simulink model "Drawing_Block"  (R2019a)
settings: Solver=VariableStepAuto  StartTime=0.0  StopTime=40  RelTol=1e-3
settings Model: Creator=Leonard  LastModifiedBy=Leonard

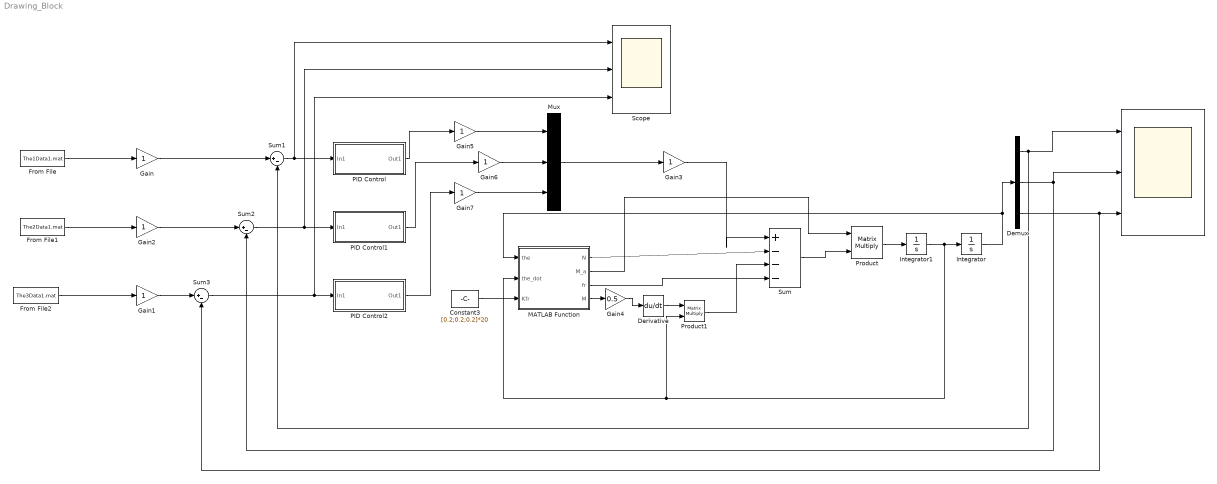
== system Drawing_Block ==
  " " : Scope  NumInputPorts=3
  Constant3 : Constant  Value=[0.2;0.2;0.2]*20
  Demux : Demux  Outputs=3
  Derivative : Derivative
  From File : FromFile  FileName=The1Data1.mat  SampleTime=0
  From File1 : FromFile  FileName=The2Data1.mat  SampleTime=0
  From File2 : FromFile  FileName=The3Data1.mat  SampleTime=0
  Gain{,1..3,5..7} (7 alike) : Gain
  Gain4 : Gain  Gain=0.5
  Integrator : Integrator  InitialCondition=[0;0;0]
  Integrator1 : Integrator  InitialCondition=[0;0;0]
  MATLAB Function : MATLAB Function  TreatAsAtomicUnit=on
  Mux : Mux  Inputs=3
  PID Control : Subsystem
  PID Control1 : Subsystem
  PID Control2 : Subsystem
  Product : Product  Multiplication=Matrix(*)
  Product1 : Product  Multiplication=Matrix(*)
  Scope : Scope  NumInputPorts=3
  Sum : Sum  Inputs=|+---
  Sum1 : Sum  Inputs=|+-
  Sum2 : Sum  Inputs=|+-
  Sum3 : Sum  Inputs=|+-
  wires:
  From File/1 -> Gain/1
  Gain6/1 -> Mux/2
  PID Control/1(Out1) -> Gain5/1
  Demux/1 -> Sum1/2, " "/1
  Demux/3 -> Sum3/2, " "/3
  Product1/1 -> Sum/3
  PID Control2/1(Out1) -> Gain7/1
  Constant3/1 -> MATLAB Function/3(Kfr)
  Gain1/1 -> Sum3/1
  Gain/1 -> Sum1/1
  PID Control1/1(Out1) -> Gain6/1
  Gain7/1 -> Mux/3
  Sum/1 -> Product/2
  Demux/2 -> " "/2, Sum2/2
  MATLAB Function/4(M) -> Gain4/1
  Gain2/1 -> Sum2/1
  From File1/1 -> Gain2/1
  Sum1/1 -> PID Control/1(In1), Scope/1
  Integrator1/1 -> Product1/2, MATLAB Function/2(the_dot), Integrator/1
  Derivative/1 -> Product1/1
  MATLAB Function/2(M_a) -> Product/1
  Sum2/1 -> PID Control1/1(In1), Scope/2
  Integrator/1 -> MATLAB Function/1(the), Demux/1
  Gain4/1 -> Derivative/1
  MATLAB Function/1(N) -> Sum/2
  MATLAB Function/3(fr) -> Sum/4
  Gain3/1 -> Sum/1
  Mux/1 -> Gain3/1
  Gain5/1 -> Mux/1
  From File2/1 -> Gain1/1
  Product/1 -> Integrator1/1
  Sum3/1 -> Scope/3, PID Control2/1(In1)

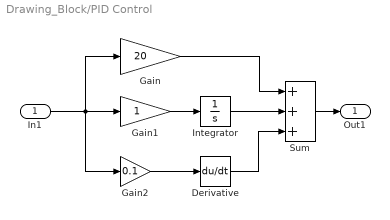
== system Drawing_Block/PID Control ==
  In1 : Inport
  Derivative : Derivative
  Gain : Gain  Gain=20
  Gain1 : Gain
  Gain2 : Gain  Gain=0.1
  Integrator : Integrator
  Sum : Sum  Inputs=+++
  Out1 : Outport
  wires:
  Sum/1 -> Out1/1
  Gain/1 -> Sum/1
  Gain2/1 -> Derivative/1
  Gain1/1 -> Integrator/1
  Integrator/1 -> Sum/2
  Derivative/1 -> Sum/3
  In1/1 -> Gain1/1, Gain2/1, Gain/1

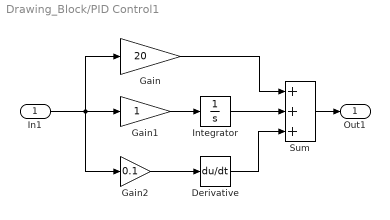
== system Drawing_Block/PID Control1 ==
  In1 : Inport
  Derivative : Derivative
  Gain : Gain  Gain=20
  Gain1 : Gain
  Gain2 : Gain  Gain=0.1
  Integrator : Integrator
  Sum : Sum  Inputs=+++
  Out1 : Outport
  wires:
  Sum/1 -> Out1/1
  Gain/1 -> Sum/1
  Gain2/1 -> Derivative/1
  Gain1/1 -> Integrator/1
  Integrator/1 -> Sum/2
  Derivative/1 -> Sum/3
  In1/1 -> Gain1/1, Gain2/1, Gain/1

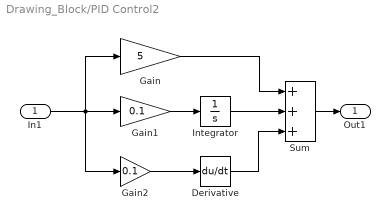
== system Drawing_Block/PID Control2 ==
  In1 : Inport
  Derivative : Derivative
  Gain : Gain  Gain=5
  Gain1 : Gain  Gain=0.1
  Gain2 : Gain  Gain=0.1
  Integrator : Integrator
  Sum : Sum  Inputs=+++
  Out1 : Outport
  wires:
  Sum/1 -> Out1/1
  Gain/1 -> Sum/1
  Gain2/1 -> Derivative/1
  Gain1/1 -> Integrator/1
  Integrator/1 -> Sum/2
  Derivative/1 -> Sum/3
  In1/1 -> Gain1/1, Gain2/1, Gain/1

== matlab function Drawing_Block/MATLAB Function ==
  data: the input; N output; M_a output; fr output; M output; the_dot input; Kfr input
function [N,M_a,fr,M] = fcn(the,the_dot,Kfr)
the1=the(1); the2=the(2); the3=the(3);
L1 = 0.2; L2 = 0.5 ; L3= 0.5; %Link length
m1 = 2 ; m2 = 0.3 ; m3 =0.1 ; %Link mass
%clc
%clear all;
%syms m1 m2 m3 L2 L3 the1 the2 the3 L1 the1_dot the2_dot the3_dot ;
%the_dot = [the1_dot; the2_dot;the3_dot];
%%%%%%%%%%%%%%%%%%%%%%%%%%%%%%%%%%%%%

%TINH JACOBIAN CHO DIEM m1
%P_0_m1 = [ 0; 0; L1];

%DAO HAM P_0_m1 THEO THE1
J_0_m1_dot_the1 = [ 0; 0; 0];
%DAO HAM P_0_m1 THEO THE2
J_0_m1_dot_the2 = [ 0; 0; 0];
%DAO HAM P_0_m1 THEO THE3
J_0_m1_dot_the3 = [ 0; 0; 0]; 

J_0_m1 = [J_0_m1_dot_the1 J_0_m1_dot_the2 J_0_m1_dot_the3];
%%%%%%%%%%%%%%%%%%%%%%%%%%%%%%%%%%%%%%%
%TINH JACOBIAN CHO DIEM m2
%P_0_m2 = [L2*cos(the1)*cos(the2); L2*cos(the2)*sin(the1); L1 + L2*sin(the2)];

%DAO HAM P_0_m2 THEO THE1
J_0_m2_dot_the1 = [L2*sin(-the1)*cos(the2);L2*cos(the2)*cos(the1); 0];
%DAO HAM P_0_m2 THEO THE2
J_0_m2_dot_the2 = [L2*cos(the1)*sin(-the2);L2*sin(-the2)*sin(the1); L2*cos(the2)];
%DAO HAM P_0_m2 THEO THE3
J_0_m2_dot_the3 = [ 0; 0; 0]; 

J_0_m2 = [J_0_m2_dot_the1  J_0_m2_dot_the2  J_0_m2_dot_the3];
%%%%%%%%%%%%%%%%%%%%%%%%%%%%%%%%%%%%%%%%%

%TINH JACOBIAN CHO DIEM m3
%P_0_m3 = [ cos(the1)*(L3*cos(the2 + the3) + L2*cos(the2)); sin(the1)*(L3*cos(the2 + the3) + L2*cos(the2)); L1 + L3*sin(the2 + the3) + L2*sin(the2)];
%DAO HAM P_0_m3 THEO THE1
J_0_m3_dot_the1 = [sin(-the1)*(L3*cos(the2 + the3) + L2*cos(the2));	 cos(the1)*(L3*cos(the2 + the3) + L2*cos(the2));     0];
%DAO HAM P_0_m3 THEO THE2
J_0_m3_dot_the2 = [cos(the1)*(L3*sin(-the2 - the3) + L2*sin(-the2));  sin(the1)*(L3*sin(-the2 - the3) + L2*sin(-the2));    L3*cos(the2 + the3) + L2*cos(the2)];
%DAO HAM P_0_m3 THEO THE3
J_0_m3_dot_the3 = [ cos(the1)*L3*sin(-the2 - the3);	 sin(the1)*L3*sin(-the2 - the3);  L3*cos(the2 + the3)];

J_0_m3 = [J_0_m3_dot_the1  J_0_m3_dot_the2  J_0_m3_dot_the3];

%%%%%%%%%%%%%%%%%%%%%%%%%%%%%%%%%%%%%%%%%%%%%%%%%%%%%%%%%%
%TONG HOP MA TRAN M3

M3 = (m3*[0 0 1]*transpose(J_0_m3)*J_0_m3)

%%%%%%%%%%%%%%%%%%%%%%%%%%%%%%%%%%%%%%%%%%%%%%%%%%%
%TONG HOP MA TRAN M2

M2 = (m2*[0 1 0]*transpose(J_0_m2)*J_0_m2 + m3*[0 1 0]*transpose(J_0_m3)*J_0_m3) 

%%%%%%%%%%%%%%%%%%%%%%%%%%%%%%%%%%%%%%%%%%%%%%%%%%%
%TONG HOP MA TRAN M1

M1 = (m1*[1 0 0]*transpose(J_0_m1)*J_0_m1 + m2*[1 0 0]*transpose(J_0_m2)*J_0_m2 + m3*[1 0 0]*transpose(J_0_m2)*J_0_m3) + [0.1 0 0];


M  = [ M1 ; M2 ; M3];
M_a = inv(M);


%%%%%%%%%%%%%%%%%%%%%%%%%%%%%%%%%%%%%%%%%%%%%%%%%%%%%%
 
%DAO HAM J_0_m1_dot_the1 theo the1

J_0_m1_dot_the1_dot_the1 = [ 0; 0; 0];
%DAO HAM J_0_m1_dot_the2 theo the1
J_0_m1_dot_the2_dot_the1 = [ 0; 0; 0];  
%DAO HAM J_0_m1_dot_the3 theo the1
J_0_m1_dot_the3_dot_the1 = [ 0; 0; 0]; 

%DAO HAM J_0_m1 theo the1 
J_0_m1_dot_the1_1 = [J_0_m1_dot_the1_dot_the1  J_0_m1_dot_the2_dot_the1  J_0_m1_dot_the3_dot_the1];

%%%%%%%%%%%%%%%%%%%%%%%%%%%%%%%%%%%%%%%%%%%%%%%%%%%%%%%%%%
%DAO HAM J_0_m2_dot_the1 theo the1
%J_0_m2_dot_the1 = [L2*sin(-the1)*cos(the2);    L2*cos(the2)*cos(the1);  0];
J_0_m2_dot_the1_dot_the1 = [L2*cos(the1)*cos(the2);L2*cos(the2)*sin(-the1); 0];
%DAO HAM J_0_m2_dot_the2 theo the1
%J_0_m2_dot_the2 = [L2*cos(the1)*sin(-the2);    L2*sin(-the2)*sin(the1);     L2*cos(the2)];
J_0_m2_dot_the2_dot_the1 = [L2*sin(the1)*sin(the2);L2*sin(-the2)*cos(the1); 0];
%DAO HAM J_0_m2_dot_the3 theo the1
J_0_m2_dot_the3_dot_the1 = [ 0; 0; 0]; 

%DAO HAM J_0_m2 theo the1 
J_0_m2_dot_the1_1 = [J_0_m2_dot_the1_dot_the1   J_0_m2_dot_the2_dot_the1  J_0_m2_dot_the3_dot_the1];

%%%%%%%%%%%%%%%%%%%%%%%%%%%%%%%%%%%%%%%%%%%%%%%%%%%%%%%%%%%
%DAO HAM J_0_m2_dot_the1 theo the2
%J_0_m2_dot_the1 = [L2*sin(-the1)*cos(the2);    L2*cos(the2)*cos(the1);  0];
J_0_m2_dot_the1_dot_the2 = [L2*sin(the1)*sin(the2);L2*sin(-the2)*cos(the1); 0];
%DAO HAM J_0_m2_dot_the2 theo the2
%J_0_m2_dot_the2 = [L2*cos(the1)*sin(-the2);    L2*sin(-the2)*sin(the1);     L2*cos(the2)];
J_0_m2_dot_the2_dot_the2 = [L2*cos(the1)*cos(the2);L2*cos(the2)*sin(the1); L2*sin(-the2)];
%DAO HAM J_0_m2_dot_the3 theo the2
J_0_m2_dot_the3_dot_the2 = [ 0; 0; 0]; 

%DAO HAM J_0_m2 theo the2
J_0_m2_dot_the2_2 = [J_0_m2_dot_the1_dot_the2  J_0_m2_dot_the2_dot_the2  J_0_m2_dot_the3_dot_the2];

%%%%%%%%%%%%%%%%%%%%%%%%%%%%%%%%%%%%%%%%%%%%%%%%%%%%%%%%%%%%%%%
%DAO HAM J_0_m3_dot_the1 theo the1
%J_0_m3_dot_the1 = [sin(-the1)*(L3*cos(the2 + the3) + L2*cos(the2));	 cos(the1)*(L3*cos(the2 + the3) + L2*cos(the2));     0];
J_0_m3_dot_the1_dot_the1 = [cos(the1)*(L3*cos(the2 + the3) + L2*cos(the2));	 sin(-the1)*(L3*cos(the2 + the3) + L2*cos(the2));     0];
%DAO HAM J_0_m3_dot_the2 theo the1
%J_0_m3_dot_the2 =          [cos(the1)*(L3*sin(-the2 - the3) + L2*sin(-the2));  sin(the1)*(L3*sin(-the2 - the3) + L2*sin(-the2));    L3*cos(the2 + the3) + L2*cos(the2)];
J_0_m3_dot_the2_dot_the1 = [sin(the1)*(L3*sin(the2 + the3) + L2*sin(the2));  -cos(the1)*(L3*sin(the2 + the3) + L2*sin(the2));    0];
%DAO HAM J_0_m3_dot_the3 theo the1
%J_0_m3_dot_the3 =          [ cos(the1)*L3*sin(-the2 - the3);	 sin(the1)*L3*sin(-the2 - the3);  L3*cos(the2 + the3)];
J_0_m3_dot_the3_dot_the1 = [ sin(the1)*L3*sin(the2 + the3);     -cos(the1)*L3*sin(the2 + the3);  0];

J_0_m3_dot_the1_1 = [J_0_m3_dot_the1_dot_the1  J_0_m3_dot_the2_dot_the1  J_0_m3_dot_the3_dot_the1];

%%%%%%%%%%%%%%%%%%%%%%%%%%%%%%%%%%%%%%%%%%%%%%%%%%%%%%%%%%%%%

%DAO HAM J_0_m3_dot_the1 theo the2
%J_0_m3_dot_the1 =          [sin(-the1)*(L3*cos(the2 + the3) + L2*cos(the2));	 cos(the1)*(L3*cos(the2 + the3) + L2*cos(the2));     0];
J_0_m3_dot_the1_dot_the2 = [sin(the1)*(L3*sin(the2 + the3) + L2*sin(the2));	 -cos(the1)*(L3*sin(the2 + the3) + L2*sin(the2));     0];
%DAO HAM J_0_m3_dot_the2 theo the2
%J_0_m3_dot_the2 =        [cos(the1)*(L3*sin(-the2 - the3) + L2*sin(-the2));  sin(the1)*(L3*sin(-the2 - the3) + L2*sin(-the2));    L3*cos(the2 + the3) + L2*cos(the2)];
J_0_m3_dot_the2_dot_the2 = [cos(the1)*(L3*cos(the2 + the3) + L2*cos(the2));  sin(the1)*(L3*cos(the2 + the3) + L2*cos(the2));    -L3*sin(the2 + the3) - L2*sin(the2)];
%DAO HAM J_0_m3_dot_the3 theo the2
%J_0_m3_dot_the3 =         [ cos(the1)*L3*sin(-the2 - the3);	 sin(the1)*L3*sin(-the2 - the3);  L3*cos(the2 + the3)];
J_0_m3_dot_the3_dot_the2 = [ cos(the1)*L3*cos(the2 + the3);     sin(the1)*L3*cos(the2 + the3);  -L3*sin(the2 + the3)];

%DAO HAM J_0_m3 theo the2
J_0_m3_dot_the2_2= [J_0_m3_dot_the1_dot_the2  J_0_m3_dot_the2_dot_the2  J_0_m3_dot_the3_dot_the2];
 

%%%%%%%%%%%%%%%%%%%%%%%%%%%%%%%%%%%%%%%%%%%%%%%%%%%%%%%%%%%%%
%DAO HAM J_0_m3_dot_the1 theo the3
%J_0_m3_dot_the1 =         [sin(-the1)*(L3*cos(the2 + the3) + L2*cos(the2));	 cos(the1)*(L3*cos(the2 + the3) + L2*cos(the2));     0];
J_0_m3_dot_the1_dot_the3 = [sin(the1)*L3*sin(the2 + the3);	 -cos(the1)*L3*sin(the2 + the3);     0];
%DAO HAM J_0_m3_dot_the2 theo the3
%J_0_m3_dot_the2 =        [cos(the1)*(L3*sin(-the2 - the3) + L2*sin(-the2));  sin(the1)*(L3*sin(-the2 - the3) + L2*sin(-the2));    L3*cos(the2 + the3) + L2*cos(the2)];
J_0_m3_dot_the2_dot_the3 = [cos(the1)*L3*cos(the2 + the3);  sin(the1)*L3*cos(the2 + the3);    -L3*sin(the2 + the3)];
%DAO HAM J_0_m3_dot_the3 theo the3
%J_0_m3_dot_the3 =         [ cos(the1)*L3*sin(-the2 - the3);	 sin(the1)*L3*sin(-the2 - the3);  L3*cos(the2 + the3)];
J_0_m3_dot_the3_dot_the3 = [ cos(the1)*L3*cos(the2 + the3);	 sin(the1)*L3*cos(the2 + the3);  -L3*sin(the2 + the3)];

%DAO HAM J_0_m3 theo the3
J_0_m3_dot_the3_3 = [J_0_m3_dot_the1_dot_the3 J_0_m3_dot_the2_dot_the3  J_0_m3_dot_the3_dot_the3];
 
%%%%%%%%%%%%%%%%%%%%%%%%%%%%%%%%%%%%%%%%%%%%%%%%%%%%%%%%%%%%%%%%%
dT_dthe3 = transpose(the_dot)*(m3*transpose(J_0_m3_dot_the3_3)*J_0_m3)*the_dot;
%%%%%%%%%%%%%%%%%%%%%%%%%%%%%%%%%%%%%%%%%%%%
dT_dthe2 = transpose(the_dot)*(m2*transpose(J_0_m2_dot_the2_2)*J_0_m2+m3*transpose(J_0_m3_dot_the2_2)*J_0_m3)*the_dot;
%%%%%%%%%%%%%%%%%%%%%%%%%%%%%%%%%%%%%%%%%%
dT_dthe1 = (transpose(the_dot)*(m1*transpose(J_0_m1_dot_the1_1)*J_0_m1+m2*transpose(J_0_m2_dot_the1_1)*J_0_m2+m3*transpose(J_0_m3_dot_the1_1)*J_0_m3)*the_dot);

%%%%%%%%%%%%%%%%%%%%%%%%%%%%%%%%%%%%%%%%%%%%%%%%%%%%%%%%%%%%%%%%%%
%M3_dot_t = [ 0,	 (L3*m3*L2*sin(-the3))*the3_dot,	 0];
%M2_dot_t = [ 0, (2*L2*L3*m3*sin(-the3))*the3_dot, 	(L3*m3*L2*sin(-the3))*the3_dot];
%M1_dot_t = [ (2*L2^2*m2*cos(the2)*sin(-the2) + 2*L2^2*m3*cos(the2)*sin(-the2) + 2*L2*L3*m3*cos(the2)*sin(-the2)*cos(the3) - L2*L3*m3*sin(-the2)*cos(the2)*sin(the3))*the2_dot + (L2*L3*m3*cos(the2)^2*sin(-the3) - L2*L3*m3*cos(the2)*sin(the2)*cos(the3))*the3_dot,	 0,	0];

%M_dot_t = [ M1_dot_t;M2_dot_t;M3_dot_t];


%%%%%%%%%%%%%%%%%%%%%%%%%%%%%%%%%%%%%%%%%%%%%%%%%%%%%%%%%
%TINH dU_DTHE3
%%%%%%%%%%%%%%%%%%%%%%%%%%%%%%%%%%%%%%%%%%%%%%%%%%%%%%%%%%%%%%%
g_0 = [ 0;0;-9.81];

dU_dthe3 = -m3*transpose(g_0)*J_0_m3_dot_the3
 
N3 = -dT_dthe3 + dU_dthe3;
%V3 = simplify(-dT_dthe3+M3_dot_t*the_dot)
%%%%%%%%%%%%%%%%%%%%%%%%%%%%%%%%%%%%%%%%%%%%%%%%%%%%%%%%%%%
%TINH dU_DTHE2
%%%%%%%%%%%%%%%%%%%%%%%%%%%%%%%%%%%%%%%%%%%%%%%%%%%%%%%%%%%%%%%
g_0 = [ 0;0;-9.81];

dU_dthe2 = -m2*transpose(g_0)*J_0_m2_dot_the2 - m3*transpose(g_0)*J_0_m3_dot_the2
 
N2= -dT_dthe2 + dU_dthe2;
%V2 = simplify(-dT_dthe2 + M2_dot_t*the_dot)
%%%%%%%%%%%%%%%%%%%%%%%%%%%%%%%%%%%%%%%%%%%%%%%%%%%%%%%%%%%
%TINH dU_DTHE1
%%%%%%%%%%%%%%%%%%%%%%%%%%%%%%%%%%%%%%%%%%%%%%%%%%%%%%%%%%%%%%%
g_0 = [ 0;0;-9.81];

dU_dthe1 = -m1*transpose(g_0)*J_0_m1_dot_the1-m2*transpose(g_0)*J_0_m2_dot_the1-m3*transpose(g_0)*J_0_m3_dot_the1
 
N1= -dT_dthe1  + dU_dthe1;
%V1 = simplify(-dT_dthe1+M1_dot_t*the_dot)
N = [ N1;N2;N3] ;
fr = [(Kfr(1)*the_dot(1)); (Kfr(2)*the_dot(2)) ; (Kfr(3)*the_dot(3))];

%%%%%%%%%%%%%%%%%%%%%%%%%%%%%%%%%%%%%%%%%%%%%%%%%%%%%%%%
%PHUONG TRINH DONG LUC HOC
%M*the_2dot + N =to
